simulink model "Manipulator_Power_Simulink1"  (R2021b)
settings: Solver=VariableStepAuto  StartTime=0.0  StopTime=10.0  RelTol=1e-3
libraries: fl_lib x72, fl_ps_legacy_lib x32, nesl_utility x24, ee_lib x8, simulink x4, slpidlib x4, simulink_extras x4
(part 2 of 2)

== system Manipulator_Power_Simulink1/JOINT2/Controller/Speed ==
  Ref : Inport  RequirementInfo={} %GIDa_133d2fbd_c93e_4f77_b4ac_eab9d76c42d5
  ERef : fl_lib/Electrical/Electrical Elements/Electrical Reference  RequirementInfo={} %GIDa_7d76ed12_3202_4e07_9a81_a49e1b94768a
  Step Rate and Direction : Subsystem  RequirementInfo={} %GIDa_caaf0cf5_7010_465f_9918_d7533aa9d66e
  Voltage-Controlled Pulse Generator : Subsystem  RequirementInfo={} %GIDa_c6184c00_e7ae_4ed6_b023_dd2e423edd06
  PWM : PMIOPort  RequirementInfo={} %GIDa_212c39cb_5b57_476e_a698_4d1e9cdd5427  Side=Right
  0v : PMIOPort  RequirementInfo={} %GIDa_c3c92952_d7df_46f2_a6c1_61685cd34345  Port=2  Side=Right
  REV : PMIOPort  RequirementInfo={} %GIDa_dc8a3b62_1286_4359_8672_6bb9b44ae351  Port=3  Side=Right
  wires:
  Ref/1 -> Step Rate and Direction/1(Reference)
  connections:
  PWM/RConn1 -- Voltage-Controlled Pulse Generator/RConn1
  Voltage-Controlled Pulse Generator/RConn2 -- 0v/RConn1 -- ERef/LConn1
  Step Rate and Direction/RConn1 -- REV/RConn1
  Step Rate and Direction/RConn2 -- Voltage-Controlled Pulse Generator/LConn1

== system Manipulator_Power_Simulink1/JOINT3/Controller/Speed ==
  Ref : Inport  RequirementInfo={} %GIDa_816022ef_432a_4a79_90a7_2ae6cbd59fcd
  ERef : fl_lib/Electrical/Electrical Elements/Electrical Reference  RequirementInfo={} %GIDa_196008e7_2150_4d1c_9562_2b404e1eb384
  Step Rate and Direction : Subsystem  RequirementInfo={} %GIDa_3dc02a5d_9463_4040_a7f9_8c5ed42feb4d
  Voltage-Controlled Pulse Generator : Subsystem  RequirementInfo={} %GIDa_cda5a4f7_7bce_4a17_92d2_0249b497aa56
  PWM : PMIOPort  RequirementInfo={} %GIDa_ae6e6dfd_0883_41b5_a79f_f2a88b9bb8a5  Side=Right
  0v : PMIOPort  RequirementInfo={} %GIDa_84d0f212_669f_417f_b7e6_49da8841d292  Port=2  Side=Right
  REV : PMIOPort  RequirementInfo={} %GIDa_363b8ad7_587b_486d_9c01_9ecb04e88f52  Port=3  Side=Right
  wires:
  Ref/1 -> Step Rate and Direction/1(Reference)
  connections:
  Step Rate and Direction/RConn2 -- Voltage-Controlled Pulse Generator/LConn1
  Step Rate and Direction/RConn1 -- REV/RConn1
  ERef/LConn1 -- 0v/RConn1 -- Voltage-Controlled Pulse Generator/RConn2
  PWM/RConn1 -- Voltage-Controlled Pulse Generator/RConn1

== system Manipulator_Power_Simulink1/JOINT4/Controller/Speed ==
  Ref : Inport  RequirementInfo={} %GIDa_d717e889_664f_4dd2_8736_eb6c370576c8
  ERef : fl_lib/Electrical/Electrical Elements/Electrical Reference  RequirementInfo={} %GIDa_8f4f37d8_c331_48d0_9e36_178249331710
  Step Rate and Direction : Subsystem  RequirementInfo={} %GIDa_7f64dba6_34d7_4fd6_b7e6_8ef2aa4dbaeb
  Voltage-Controlled Pulse Generator : Subsystem  RequirementInfo={} %GIDa_cf4eb0bf_28be_416a_a242_a03039ffa540
  PWM : PMIOPort  RequirementInfo={} %GIDa_aef454f5_c686_4161_86a7_873aeed7fd4b  Side=Right
  0v : PMIOPort  RequirementInfo={} %GIDa_3be3be1f_d3f7_46ea_ae96_b67254762afc  Port=2  Side=Right
  REV : PMIOPort  RequirementInfo={} %GIDa_ffa23ca5_42c1_4813_9242_4a9203d3890b  Port=3  Side=Right
  wires:
  Ref/1 -> Step Rate and Direction/1(Reference)
  connections:
  PWM/RConn1 -- Voltage-Controlled Pulse Generator/RConn1
  Voltage-Controlled Pulse Generator/RConn2 -- 0v/RConn1 -- ERef/LConn1
  Step Rate and Direction/RConn1 -- REV/RConn1
  Step Rate and Direction/RConn2 -- Voltage-Controlled Pulse Generator/LConn1

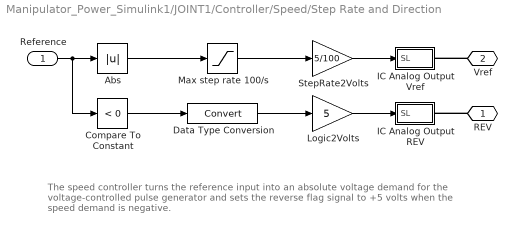
== system Manipulator_Power_Simulink1/JOINT1/Controller/Speed/Step Rate and Direction ==
  note: The speed controller turns the reference input into an absolute voltage demand for the
      | voltage-controlled pulse generator and sets the reverse flag signal to +5 volts when the
      | speed demand is negative.
  Reference : Inport  RequirementInfo={} %GIDa_a4d0a8f3_775c_42b8_9ce6_c57082dd7fd6
  Abs : Abs  RequirementInfo={} %GIDa_7613da56_6ee1_41bb_bf24_79eccb83e254
  Compare To Constant : simulink/Logic and Bit Operations/Compare To Constant  relop=<  const=0  OutDataTypeStr=uint8  ZeroCross=off
  Data Type Conversion : DataTypeConversion  RequirementInfo={} %GIDa_15417bf0_c7ec_4a8f_8ffd_c88ebbfd43ea
  IC Analog Output REV : Subsystem  RequirementInfo={} %GIDa_2381db1b_a9cd_4814_b69d_fad528507182
  IC Analog Output Vref : Subsystem  RequirementInfo={} %GIDa_7a2ed817_81c4_46ea_bee9_8975aad226ea
  Logic2Volts : Gain  RequirementInfo={} %GIDa_359c6216_a839_4c16_a394_d78c702d9162  Gain=5
  Max step rate 100/s : Saturate  RequirementInfo={} %GIDa_432da2a1_418c_4d16_83eb_56a19b9fecce  UpperLimit=100  LowerLimit=0
  StepRate2Volts : Gain  RequirementInfo={} %GIDa_aa390892_47b5_48bb_8fe1_8b1239142bf5  Gain=5/100
  REV : PMIOPort  RequirementInfo={} %GIDa_b21a2a82_f1de_4c93_a224_afadd27e55c2  Side=Right
  Vref : PMIOPort  RequirementInfo={} %GIDa_5a2899ae_9d44_4071_a42f_9f02a65277c8  Port=2  Side=Right
  wires:
  Logic2Volts/1 -> IC Analog Output REV/1(SL)
  Abs/1 -> Max step rate 100/s/1
  Reference/1 -> Abs/1, Compare To Constant/1
  Compare To Constant/1 -> Data Type Conversion/1
  Data Type Conversion/1 -> Logic2Volts/1
  Max step rate 100/s/1 -> StepRate2Volts/1
  StepRate2Volts/1 -> IC Analog Output Vref/1(SL)
  connections:
  Vref/RConn1 -- IC Analog Output Vref/RConn1
  REV/RConn1 -- IC Analog Output REV/RConn1

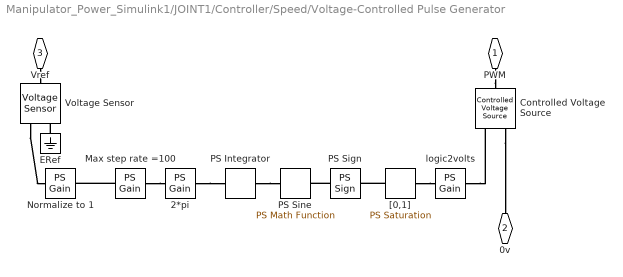
== system Manipulator_Power_Simulink1/JOINT1/Controller/Speed/Voltage-Controlled Pulse Generator ==
  2*pi : fl_ps_legacy_lib/Legacy Physical Signals/Functions/PS Gain  RequirementInfo={} %GIDa_61df0c9e_b235_4c70_930a_adc0727db65f  gain=-2*pi
  Controlled Voltage Source : fl_lib/Electrical/Electrical Sources/Controlled Voltage Source  RequirementInfo={} %GIDa_890246c1_4e7d_432c_91b9_002d9def5f11
  ERef : fl_lib/Electrical/Electrical Elements/Electrical Reference  RequirementInfo={} %GIDa_3d71df36_8a4a_4c67_937d_640ca4b360d2
  Max step rate =100 : fl_ps_legacy_lib/Legacy Physical Signals/Functions/PS Gain  RequirementInfo={} %GIDa_eb934f0b_f6ff_49ce_bc85_53990e09ede5  gain=100
  Normalize to 1 : fl_ps_legacy_lib/Legacy Physical Signals/Functions/PS Gain  RequirementInfo={} %GIDa_5c71ac23_9195_42cc_b2ed_1502285f8c0f  gain=1/5
  PS Integrator : fl_ps_legacy_lib/Legacy Physical Signals/Linear Operators/PS Integrator  RequirementInfo={} %GIDa_2c83dace_df5d_4329_b79b_3a0dcf4e6b2a  x0=0
      settings: SourceProductBaseCode=SS  InternalSimscapePortConfiguration="{\"Bottom\":[],\"Left\":[{\"id\":\"I\",\"label\":\"\",\"type\":\"input\"}],\"Right\":[{\"id\":\"O\",\"label\":\"\",\"type\":\"output\"}],\"Top\":[]}"
  PS Sign : fl_ps_legacy_lib/Legacy Physical Signals/Nonlinear Operators/PS Sign  RequirementInfo={} %GIDa_f0cac072_c839_41db_b2f7_6ab4e4664324
      settings: SourceProductBaseCode=SS  InternalSimscapePortConfiguration="{\"Bottom\":[],\"Left\":[{\"id\":\"I\",\"label\":\"\",\"type\":\"input\"}],\"Right\":[{\"id\":\"O\",\"label\":\"\",\"type\":\"output\"}],\"Top\":[]}"
  PS Sine : fl_ps_legacy_lib/Legacy Physical Signals/Functions/PS Math Function  RequirementInfo={} %GIDa_6e5c4b4c_1fe3_442e_b21e_5b744a8abd76  fcn_choice=1
      settings: SourceProductBaseCode=SS  InternalSimscapePortConfiguration="{\"Bottom\":[],\"Left\":[{\"id\":\"I\",\"label\":\"\",\"type\":\"input\"}],\"Right\":[{\"id\":\"O\",\"label\":\"\",\"type\":\"output\"}],\"Top\":[]}"
  Voltage Sensor : fl_lib/Electrical/Electrical Sensors/Voltage Sensor  RequirementInfo={} %GIDa_a373e7ac_be28_43af_8d8c_244c39e826c1
  "[0,1]" : fl_ps_legacy_lib/Legacy Physical Signals/Nonlinear Operators/PS Saturation  RequirementInfo={} %GIDa_5495923a_3b44_4237_bdb7_0f954ea1e40d  upper_limit=1  lower_limit=0
      settings: SourceProductBaseCode=SS  InternalSimscapePortConfiguration="{\"Bottom\":[],\"Left\":[{\"id\":\"I\",\"label\":\"\",\"type\":\"input\"}],\"Right\":[{\"id\":\"O\",\"label\":\"\",\"type\":\"output\"}],\"Top\":[]}"
  logic2volts : fl_ps_legacy_lib/Legacy Physical Signals/Functions/PS Gain  RequirementInfo={} %GIDa_083ec3bc_2847_48bb_b782_91084d8168f5  gain=5
  PWM : PMIOPort  RequirementInfo={} %GIDa_4cd06a5c_1eea_49eb_bdb7_282e6aefe270  Side=Right
  0v : PMIOPort  RequirementInfo={} %GIDa_96d2d6b6_c14e_4d63_87b4_9d47c63deab9  Port=2  Side=Right
  Vref : PMIOPort  RequirementInfo={} %GIDa_2a267a3e_713f_4133_af62_9dc00d10e885  Port=3  Side=Left
  connections:
  logic2volts/RConn1 -- Controlled Voltage Source/RConn1
  "[0,1]"/RConn1 -- logic2volts/LConn1
  "[0,1]"/LConn1 -- PS Sign/RConn1
  PS Sign/LConn1 -- PS Sine/RConn1
  PS Integrator/RConn1 -- PS Sine/LConn1
  2*pi/RConn1 -- PS Integrator/LConn1
  Max step rate =100/RConn1 -- 2*pi/LConn1
  Max step rate =100/LConn1 -- Normalize to 1/RConn1
  Voltage Sensor/RConn1 -- Normalize to 1/LConn1
  ERef/LConn1 -- Voltage Sensor/RConn2
  Vref/RConn1 -- Voltage Sensor/LConn1
  Controlled Voltage Source/RConn2 -- 0v/RConn1
  PWM/RConn1 -- Controlled Voltage Source/LConn1

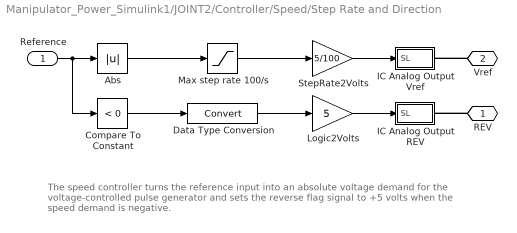
== system Manipulator_Power_Simulink1/JOINT2/Controller/Speed/Step Rate and Direction ==
  note: The speed controller turns the reference input into an absolute voltage demand for the
      | voltage-controlled pulse generator and sets the reverse flag signal to +5 volts when the
      | speed demand is negative.
  Reference : Inport  RequirementInfo={} %GIDa_90aba829_d451_4a5e_aa85_55f83649f4db
  Abs : Abs  RequirementInfo={} %GIDa_c9b203d5_6184_4a9d_ad90_f83fc17c6376
  Compare To Constant : simulink/Logic and Bit Operations/Compare To Constant  relop=<  const=0  OutDataTypeStr=uint8  ZeroCross=off
  Data Type Conversion : DataTypeConversion  RequirementInfo={} %GIDa_43c8ecc9_fa97_4981_9627_7cee22fda550
  IC Analog Output REV : Subsystem  RequirementInfo={} %GIDa_ece9aa21_0efe_49d4_b00f_8f3649ea2b46
  IC Analog Output Vref : Subsystem  RequirementInfo={} %GIDa_c052096d_f211_49fe_bd90_0695814d8abb
  Logic2Volts : Gain  RequirementInfo={} %GIDa_66d68ea1_9468_4636_a012_2b3722893939  Gain=5
  Max step rate 100/s : Saturate  RequirementInfo={} %GIDa_e4ccdf5f_c923_46ec_be92_c720fdfcfe89  UpperLimit=100  LowerLimit=0
  StepRate2Volts : Gain  RequirementInfo={} %GIDa_d1820e5c_7501_48ce_a768_ecf098b9c526  Gain=5/100
  REV : PMIOPort  RequirementInfo={} %GIDa_0581cefe_2bd8_489e_9052_9096d03c1b9a  Side=Right
  Vref : PMIOPort  RequirementInfo={} %GIDa_241c3493_720f_4f49_b456_999d10fd9f84  Port=2  Side=Right
  wires:
  StepRate2Volts/1 -> IC Analog Output Vref/1(SL)
  Max step rate 100/s/1 -> StepRate2Volts/1
  Data Type Conversion/1 -> Logic2Volts/1
  Compare To Constant/1 -> Data Type Conversion/1
  Reference/1 -> Compare To Constant/1, Abs/1
  Abs/1 -> Max step rate 100/s/1
  Logic2Volts/1 -> IC Analog Output REV/1(SL)
  connections:
  REV/RConn1 -- IC Analog Output REV/RConn1
  Vref/RConn1 -- IC Analog Output Vref/RConn1

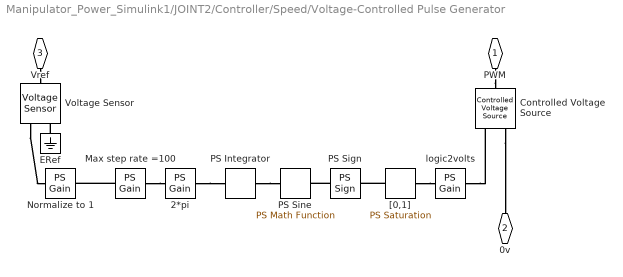
== system Manipulator_Power_Simulink1/JOINT2/Controller/Speed/Voltage-Controlled Pulse Generator ==
  2*pi : fl_ps_legacy_lib/Legacy Physical Signals/Functions/PS Gain  RequirementInfo={} %GIDa_39e0f13f_ed03_40b4_bff0_704818bbd013  gain=-2*pi
  Controlled Voltage Source : fl_lib/Electrical/Electrical Sources/Controlled Voltage Source  RequirementInfo={} %GIDa_3f254ddd_a112_40da_8740_ab4ae00e6674
  ERef : fl_lib/Electrical/Electrical Elements/Electrical Reference  RequirementInfo={} %GIDa_aa12cf46_d350_4702_8bd6_c00e57a06f4e
  Max step rate =100 : fl_ps_legacy_lib/Legacy Physical Signals/Functions/PS Gain  RequirementInfo={} %GIDa_0262f2d3_1b67_4f1f_8188_fa8785035f93  gain=100
  Normalize to 1 : fl_ps_legacy_lib/Legacy Physical Signals/Functions/PS Gain  RequirementInfo={} %GIDa_8dc38732_8c04_47cc_b45a_cab155dda67b  gain=1/5
  PS Integrator : fl_ps_legacy_lib/Legacy Physical Signals/Linear Operators/PS Integrator  RequirementInfo={} %GIDa_51806525_f935_4d2f_8466_5852c52c21b4  x0=0
      settings: SourceProductBaseCode=SS  InternalSimscapePortConfiguration="{\"Bottom\":[],\"Left\":[{\"id\":\"I\",\"label\":\"\",\"type\":\"input\"}],\"Right\":[{\"id\":\"O\",\"label\":\"\",\"type\":\"output\"}],\"Top\":[]}"
  PS Sign : fl_ps_legacy_lib/Legacy Physical Signals/Nonlinear Operators/PS Sign  RequirementInfo={} %GIDa_979e4ac6_6728_4e81_892d_596687daac1f
      settings: SourceProductBaseCode=SS  InternalSimscapePortConfiguration="{\"Bottom\":[],\"Left\":[{\"id\":\"I\",\"label\":\"\",\"type\":\"input\"}],\"Right\":[{\"id\":\"O\",\"label\":\"\",\"type\":\"output\"}],\"Top\":[]}"
  PS Sine : fl_ps_legacy_lib/Legacy Physical Signals/Functions/PS Math Function  RequirementInfo={} %GIDa_d7491fba_bca0_4560_8f49_912ad2ea4dc1  fcn_choice=1
      settings: SourceProductBaseCode=SS  InternalSimscapePortConfiguration="{\"Bottom\":[],\"Left\":[{\"id\":\"I\",\"label\":\"\",\"type\":\"input\"}],\"Right\":[{\"id\":\"O\",\"label\":\"\",\"type\":\"output\"}],\"Top\":[]}"
  Voltage Sensor : fl_lib/Electrical/Electrical Sensors/Voltage Sensor  RequirementInfo={} %GIDa_d2de3142_6796_463e_b13f_d7b525af65fd
  "[0,1]" : fl_ps_legacy_lib/Legacy Physical Signals/Nonlinear Operators/PS Saturation  RequirementInfo={} %GIDa_2a538ce2_d55b_4ca7_b3f2_8996148affe4  upper_limit=1  lower_limit=0
      settings: SourceProductBaseCode=SS  InternalSimscapePortConfiguration="{\"Bottom\":[],\"Left\":[{\"id\":\"I\",\"label\":\"\",\"type\":\"input\"}],\"Right\":[{\"id\":\"O\",\"label\":\"\",\"type\":\"output\"}],\"Top\":[]}"
  logic2volts : fl_ps_legacy_lib/Legacy Physical Signals/Functions/PS Gain  RequirementInfo={} %GIDa_1da96181_0729_44e5_ab12_b3f446b1ef09  gain=5
  PWM : PMIOPort  RequirementInfo={} %GIDa_5ea3616d_b8a3_4cc2_9d21_4ee89ba264a6  Side=Right
  0v : PMIOPort  RequirementInfo={} %GIDa_217c9688_de14_4ae3_9fb7_afb5736173ab  Port=2  Side=Right
  Vref : PMIOPort  RequirementInfo={} %GIDa_a8697067_ee00_4349_a0d9_3a9618a53fc4  Port=3  Side=Left
  connections:
  PWM/RConn1 -- Controlled Voltage Source/LConn1
  Controlled Voltage Source/RConn2 -- 0v/RConn1
  Vref/RConn1 -- Voltage Sensor/LConn1
  ERef/LConn1 -- Voltage Sensor/RConn2
  Voltage Sensor/RConn1 -- Normalize to 1/LConn1
  Max step rate =100/LConn1 -- Normalize to 1/RConn1
  Max step rate =100/RConn1 -- 2*pi/LConn1
  2*pi/RConn1 -- PS Integrator/LConn1
  PS Integrator/RConn1 -- PS Sine/LConn1
  PS Sign/LConn1 -- PS Sine/RConn1
  "[0,1]"/LConn1 -- PS Sign/RConn1
  "[0,1]"/RConn1 -- logic2volts/LConn1
  logic2volts/RConn1 -- Controlled Voltage Source/RConn1

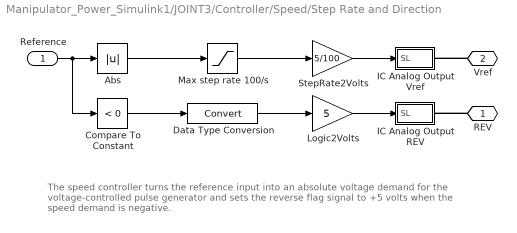
== system Manipulator_Power_Simulink1/JOINT3/Controller/Speed/Step Rate and Direction ==
  note: The speed controller turns the reference input into an absolute voltage demand for the
      | voltage-controlled pulse generator and sets the reverse flag signal to +5 volts when the
      | speed demand is negative.
  Reference : Inport  RequirementInfo={} %GIDa_e41558cf_4cf6_4664_8058_0312b625df14
  Abs : Abs  RequirementInfo={} %GIDa_35eed948_d26b_445f_bafd_d904c0444c28
  Compare To Constant : simulink/Logic and Bit Operations/Compare To Constant  relop=<  const=0  OutDataTypeStr=uint8  ZeroCross=off
  Data Type Conversion : DataTypeConversion  RequirementInfo={} %GIDa_c55a0244_950d_4825_8ab4_38179d1a507b
  IC Analog Output REV : Subsystem  RequirementInfo={} %GIDa_b1afa9ee_bd98_4eaf_a4b6_2b4cd345befe
  IC Analog Output Vref : Subsystem  RequirementInfo={} %GIDa_dc1860ae_6cf6_4062_b3c0_bc69cd577efa
  Logic2Volts : Gain  RequirementInfo={} %GIDa_797ab312_e620_4b9d_a3cb_83908b24325f  Gain=5
  Max step rate 100/s : Saturate  RequirementInfo={} %GIDa_b28a9105_40d4_4f94_b332_87ddbf6cc823  UpperLimit=100  LowerLimit=0
  StepRate2Volts : Gain  RequirementInfo={} %GIDa_33a0acae_85f0_4059_9e4d_70e14c1e9ee0  Gain=5/100
  REV : PMIOPort  RequirementInfo={} %GIDa_933b063f_5666_4fd7_a8e4_d5d0fda9cf01  Side=Right
  Vref : PMIOPort  RequirementInfo={} %GIDa_5cb1fd0e_612c_4f03_ad27_996cba0e183e  Port=2  Side=Right
  wires:
  Logic2Volts/1 -> IC Analog Output REV/1(SL)
  Abs/1 -> Max step rate 100/s/1
  Reference/1 -> Abs/1, Compare To Constant/1
  Compare To Constant/1 -> Data Type Conversion/1
  Data Type Conversion/1 -> Logic2Volts/1
  Max step rate 100/s/1 -> StepRate2Volts/1
  StepRate2Volts/1 -> IC Analog Output Vref/1(SL)
  connections:
  Vref/RConn1 -- IC Analog Output Vref/RConn1
  REV/RConn1 -- IC Analog Output REV/RConn1

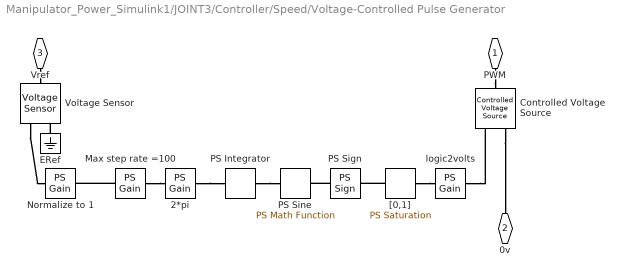
== system Manipulator_Power_Simulink1/JOINT3/Controller/Speed/Voltage-Controlled Pulse Generator ==
  2*pi : fl_ps_legacy_lib/Legacy Physical Signals/Functions/PS Gain  RequirementInfo={} %GIDa_b740e3cc_25e5_4f30_a797_9c6ce1231883  gain=-2*pi
  Controlled Voltage Source : fl_lib/Electrical/Electrical Sources/Controlled Voltage Source  RequirementInfo={} %GIDa_79ae19dc_ab4d_4dc5_8ad2_a3820feb6f8a
  ERef : fl_lib/Electrical/Electrical Elements/Electrical Reference  RequirementInfo={} %GIDa_a7b81ec0_8f1c_4f37_946e_7c8db6e35412
  Max step rate =100 : fl_ps_legacy_lib/Legacy Physical Signals/Functions/PS Gain  RequirementInfo={} %GIDa_9cbbd355_74fa_4684_bd10_e89996d8b818  gain=100
  Normalize to 1 : fl_ps_legacy_lib/Legacy Physical Signals/Functions/PS Gain  RequirementInfo={} %GIDa_6a0b4414_d6fe_414b_a7ee_e9952919e3b0  gain=1/5
  PS Integrator : fl_ps_legacy_lib/Legacy Physical Signals/Linear Operators/PS Integrator  RequirementInfo={} %GIDa_861ac414_fd0d_4e43_aab2_71d62cf93405  x0=0
      settings: SourceProductBaseCode=SS  InternalSimscapePortConfiguration="{\"Bottom\":[],\"Left\":[{\"id\":\"I\",\"label\":\"\",\"type\":\"input\"}],\"Right\":[{\"id\":\"O\",\"label\":\"\",\"type\":\"output\"}],\"Top\":[]}"
  PS Sign : fl_ps_legacy_lib/Legacy Physical Signals/Nonlinear Operators/PS Sign  RequirementInfo={} %GIDa_0be84da2_46c6_4942_8052_a17cc1d925c5
      settings: SourceProductBaseCode=SS  InternalSimscapePortConfiguration="{\"Bottom\":[],\"Left\":[{\"id\":\"I\",\"label\":\"\",\"type\":\"input\"}],\"Right\":[{\"id\":\"O\",\"label\":\"\",\"type\":\"output\"}],\"Top\":[]}"
  PS Sine : fl_ps_legacy_lib/Legacy Physical Signals/Functions/PS Math Function  RequirementInfo={} %GIDa_7faa4cb9_08e4_49ad_90c8_4ace7a404225  fcn_choice=1
      settings: SourceProductBaseCode=SS  InternalSimscapePortConfiguration="{\"Bottom\":[],\"Left\":[{\"id\":\"I\",\"label\":\"\",\"type\":\"input\"}],\"Right\":[{\"id\":\"O\",\"label\":\"\",\"type\":\"output\"}],\"Top\":[]}"
  Voltage Sensor : fl_lib/Electrical/Electrical Sensors/Voltage Sensor  RequirementInfo={} %GIDa_17c2efd4_9685_4d35_9a32_364b52e641a9
  "[0,1]" : fl_ps_legacy_lib/Legacy Physical Signals/Nonlinear Operators/PS Saturation  RequirementInfo={} %GIDa_279308bb_61ee_4a77_99bb_4cc027ccbb41  upper_limit=1  lower_limit=0
      settings: SourceProductBaseCode=SS  InternalSimscapePortConfiguration="{\"Bottom\":[],\"Left\":[{\"id\":\"I\",\"label\":\"\",\"type\":\"input\"}],\"Right\":[{\"id\":\"O\",\"label\":\"\",\"type\":\"output\"}],\"Top\":[]}"
  logic2volts : fl_ps_legacy_lib/Legacy Physical Signals/Functions/PS Gain  RequirementInfo={} %GIDa_2e4f5c9e_e808_4ed4_bda1_44483ff0252e  gain=5
  PWM : PMIOPort  RequirementInfo={} %GIDa_0ffd18b3_a9dd_40a7_b8a8_1eb886078c4b  Side=Right
  0v : PMIOPort  RequirementInfo={} %GIDa_ebf6917d_3fbc_409e_92ca_a4843bad0fc7  Port=2  Side=Right
  Vref : PMIOPort  RequirementInfo={} %GIDa_eb93b3dc_32ae_432d_9f8e_911f11189326  Port=3  Side=Left
  connections:
  logic2volts/RConn1 -- Controlled Voltage Source/RConn1
  "[0,1]"/RConn1 -- logic2volts/LConn1
  "[0,1]"/LConn1 -- PS Sign/RConn1
  PS Sign/LConn1 -- PS Sine/RConn1
  PS Integrator/RConn1 -- PS Sine/LConn1
  2*pi/RConn1 -- PS Integrator/LConn1
  Max step rate =100/RConn1 -- 2*pi/LConn1
  Max step rate =100/LConn1 -- Normalize to 1/RConn1
  Voltage Sensor/RConn1 -- Normalize to 1/LConn1
  ERef/LConn1 -- Voltage Sensor/RConn2
  Vref/RConn1 -- Voltage Sensor/LConn1
  Controlled Voltage Source/RConn2 -- 0v/RConn1
  PWM/RConn1 -- Controlled Voltage Source/LConn1

== system Manipulator_Power_Simulink1/JOINT4/Controller/Speed/Step Rate and Direction ==
  note: The speed controller turns the reference input into an absolute voltage demand for the
      | voltage-controlled pulse generator and sets the reverse flag signal to +5 volts when the
      | speed demand is negative.
  Reference : Inport  RequirementInfo={} %GIDa_3c1cf7f4_8aab_4b27_a15c_4f3445e2c108
  Abs : Abs  RequirementInfo={} %GIDa_a4c5ff9f_f4bc_4419_b386_0b71cd9cee93
  Compare To Constant : simulink/Logic and Bit Operations/Compare To Constant  relop=<  const=0  OutDataTypeStr=uint8  ZeroCross=off
  Data Type Conversion : DataTypeConversion  RequirementInfo={} %GIDa_4f1de8ed_cf8e_4042_831c_225004c8baf2
  IC Analog Output REV : Subsystem  RequirementInfo={} %GIDa_5777efa7_63e1_4053_84f0_4436bc30bc7b
  IC Analog Output Vref : Subsystem  RequirementInfo={} %GIDa_a7a73a31_6963_4ebd_8f5f_7274d19066b4
  Logic2Volts : Gain  RequirementInfo={} %GIDa_5f42dbbb_8cbc_46eb_b421_9f975a17c297  Gain=5
  Max step rate 100/s : Saturate  RequirementInfo={} %GIDa_95e6a340_9705_4d91_b485_31b055d80ecd  UpperLimit=100  LowerLimit=0
  StepRate2Volts : Gain  RequirementInfo={} %GIDa_b37e94c9_8c2e_41ef_a5c1_e1e9e4ddc3ce  Gain=5/100
  REV : PMIOPort  RequirementInfo={} %GIDa_7dc94042_af75_405a_a6d0_8ac37ce84735  Side=Right
  Vref : PMIOPort  RequirementInfo={} %GIDa_2d157ce9_f094_4672_bc4f_925f4b8a320b  Port=2  Side=Right
  wires:
  StepRate2Volts/1 -> IC Analog Output Vref/1(SL)
  Max step rate 100/s/1 -> StepRate2Volts/1
  Data Type Conversion/1 -> Logic2Volts/1
  Compare To Constant/1 -> Data Type Conversion/1
  Reference/1 -> Compare To Constant/1, Abs/1
  Abs/1 -> Max step rate 100/s/1
  Logic2Volts/1 -> IC Analog Output REV/1(SL)
  connections:
  REV/RConn1 -- IC Analog Output REV/RConn1
  Vref/RConn1 -- IC Analog Output Vref/RConn1

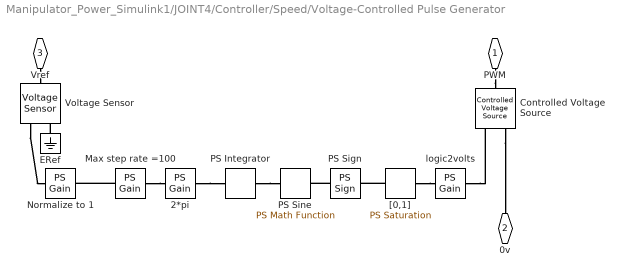
== system Manipulator_Power_Simulink1/JOINT4/Controller/Speed/Voltage-Controlled Pulse Generator ==
  2*pi : fl_ps_legacy_lib/Legacy Physical Signals/Functions/PS Gain  RequirementInfo={} %GIDa_66813b41_8fd0_4aca_b763_be0e326a44b9  gain=-2*pi
  Controlled Voltage Source : fl_lib/Electrical/Electrical Sources/Controlled Voltage Source  RequirementInfo={} %GIDa_65cba9e0_ee6d_4148_b9d1_3429b3ec2b17
  ERef : fl_lib/Electrical/Electrical Elements/Electrical Reference  RequirementInfo={} %GIDa_cddc951d_b424_40ff_9103_14f4b3e43b41
  Max step rate =100 : fl_ps_legacy_lib/Legacy Physical Signals/Functions/PS Gain  RequirementInfo={} %GIDa_ba40341b_bcb9_408b_afc4_04d5e290f9fe  gain=100
  Normalize to 1 : fl_ps_legacy_lib/Legacy Physical Signals/Functions/PS Gain  RequirementInfo={} %GIDa_5d235928_9757_4d05_9898_0539ebf6ac7e  gain=1/5
  PS Integrator : fl_ps_legacy_lib/Legacy Physical Signals/Linear Operators/PS Integrator  RequirementInfo={} %GIDa_46c26e47_d25d_4678_9c77_a70f260d309f  x0=0
      settings: SourceProductBaseCode=SS  InternalSimscapePortConfiguration="{\"Bottom\":[],\"Left\":[{\"id\":\"I\",\"label\":\"\",\"type\":\"input\"}],\"Right\":[{\"id\":\"O\",\"label\":\"\",\"type\":\"output\"}],\"Top\":[]}"
  PS Sign : fl_ps_legacy_lib/Legacy Physical Signals/Nonlinear Operators/PS Sign  RequirementInfo={} %GIDa_90bbde27_a939_4f52_8f32_954059597cda
      settings: SourceProductBaseCode=SS  InternalSimscapePortConfiguration="{\"Bottom\":[],\"Left\":[{\"id\":\"I\",\"label\":\"\",\"type\":\"input\"}],\"Right\":[{\"id\":\"O\",\"label\":\"\",\"type\":\"output\"}],\"Top\":[]}"
  PS Sine : fl_ps_legacy_lib/Legacy Physical Signals/Functions/PS Math Function  RequirementInfo={} %GIDa_fe48fc95_b233_4a8d_92fb_2e7595bfc7f9  fcn_choice=1
      settings: SourceProductBaseCode=SS  InternalSimscapePortConfiguration="{\"Bottom\":[],\"Left\":[{\"id\":\"I\",\"label\":\"\",\"type\":\"input\"}],\"Right\":[{\"id\":\"O\",\"label\":\"\",\"type\":\"output\"}],\"Top\":[]}"
  Voltage Sensor : fl_lib/Electrical/Electrical Sensors/Voltage Sensor  RequirementInfo={} %GIDa_f6a543b8_fe6d_4c52_ba0d_d5dd69f7b865
  "[0,1]" : fl_ps_legacy_lib/Legacy Physical Signals/Nonlinear Operators/PS Saturation  RequirementInfo={} %GIDa_c0b3b3c9_3657_471f_ac15_3fc2c11f2843  upper_limit=1  lower_limit=0
      settings: SourceProductBaseCode=SS  InternalSimscapePortConfiguration="{\"Bottom\":[],\"Left\":[{\"id\":\"I\",\"label\":\"\",\"type\":\"input\"}],\"Right\":[{\"id\":\"O\",\"label\":\"\",\"type\":\"output\"}],\"Top\":[]}"
  logic2volts : fl_ps_legacy_lib/Legacy Physical Signals/Functions/PS Gain  RequirementInfo={} %GIDa_8f360269_0cb4_481d_b6f5_c992905e9f39  gain=5
  PWM : PMIOPort  RequirementInfo={} %GIDa_6e010553_9f83_4703_a732_cd3f866b258e  Side=Right
  0v : PMIOPort  RequirementInfo={} %GIDa_cfc93a1d_2cc5_43ca_af35_a8fdc155dd0d  Port=2  Side=Right
  Vref : PMIOPort  RequirementInfo={} %GIDa_330d7adb_35be_4f9a_92d8_c21dff02abe9  Port=3  Side=Left
  connections:
  PWM/RConn1 -- Controlled Voltage Source/LConn1
  Controlled Voltage Source/RConn2 -- 0v/RConn1
  Vref/RConn1 -- Voltage Sensor/LConn1
  ERef/LConn1 -- Voltage Sensor/RConn2
  Voltage Sensor/RConn1 -- Normalize to 1/LConn1
  Max step rate =100/LConn1 -- Normalize to 1/RConn1
  Max step rate =100/RConn1 -- 2*pi/LConn1
  2*pi/RConn1 -- PS Integrator/LConn1
  PS Integrator/RConn1 -- PS Sine/LConn1
  PS Sign/LConn1 -- PS Sine/RConn1
  "[0,1]"/LConn1 -- PS Sign/RConn1
  "[0,1]"/RConn1 -- logic2volts/LConn1
  logic2volts/RConn1 -- Controlled Voltage Source/RConn1

== system Manipulator_Power_Simulink1/JOINT1/Controller/Speed/Step Rate and Direction/IC Analog Output REV ==
  SL : Inport  RequirementInfo={} %GIDa_02c26200_b0a8_4d42_bf0d_0515453987ae
  Controlled Voltage Source : fl_lib/Electrical/Electrical Sources/Controlled Voltage Source  RequirementInfo={} %GIDa_0c5eaec1_3691_4fd4_aa27_3131dd8f70af
  ERef : fl_lib/Electrical/Electrical Elements/Electrical Reference  RequirementInfo={} %GIDa_7b4c6f4b_a7ad_4dd6_b0e2_f0e6e1e68a66
  Simulink-PS Converter : nesl_utility/Simulink-PS Converter  RequirementInfo={} %GIDa_24446364_eec0_4d48_8623_babd559e7409  PhysicalDomain=network_engine_domain  SubClassName=ps_input  LeftPortType=input  RightPortType=output  PseudoPeriodic=off  Frequencies=[]  NoiseDistribution=none  NoiseParameters=[]  Unit=V  AffineConversion=off  FilteringAndDerivatives=zero  SimscapeFilterOrder=1  InputFilterTimeConstant=.001  UdotUserProvided=0
      settings: SourceProductBaseCode=PW,SS
  V : PMIOPort  RequirementInfo={} %GIDa_c38a79aa_0966_4c84_b0e1_9462a22e10f8  Side=Right
  wires:
  SL/1 -> Simulink-PS Converter/1
  connections:
  ERef/LConn1 -- Controlled Voltage Source/RConn2
  V/RConn1 -- Controlled Voltage Source/LConn1
  Simulink-PS Converter/RConn1 -- Controlled Voltage Source/RConn1

== system Manipulator_Power_Simulink1/JOINT1/Controller/Speed/Step Rate and Direction/IC Analog Output Vref ==
  SL : Inport  RequirementInfo={} %GIDa_f1190acc_3ebd_43d4_99b6_97e9d6f492b0
  Controlled Voltage Source : fl_lib/Electrical/Electrical Sources/Controlled Voltage Source  RequirementInfo={} %GIDa_8b110c0c_63b4_4b21_950a_268b6b8bab3d
  ERef : fl_lib/Electrical/Electrical Elements/Electrical Reference  RequirementInfo={} %GIDa_b02017e9_721d_4b2d_986b_adb6afa2a9d3
  Simulink-PS Converter : nesl_utility/Simulink-PS Converter  RequirementInfo={} %GIDa_e31afa12_1f43_4fe4_975f_f7db0b5afe35  PhysicalDomain=network_engine_domain  SubClassName=ps_input  LeftPortType=input  RightPortType=output  PseudoPeriodic=off  Frequencies=[]  NoiseDistribution=none  NoiseParameters=[]  Unit=V  AffineConversion=off  FilteringAndDerivatives=zero  SimscapeFilterOrder=1  InputFilterTimeConstant=.001  UdotUserProvided=0
      settings: SourceProductBaseCode=PW,SS
  V : PMIOPort  RequirementInfo={} %GIDa_7fc42ce3_83a4_46fe_bd47_de0850ef379b  Side=Right
  wires:
  SL/1 -> Simulink-PS Converter/1
  connections:
  Simulink-PS Converter/RConn1 -- Controlled Voltage Source/RConn1
  V/RConn1 -- Controlled Voltage Source/LConn1
  ERef/LConn1 -- Controlled Voltage Source/RConn2

== system Manipulator_Power_Simulink1/JOINT2/Controller/Speed/Step Rate and Direction/IC Analog Output REV ==
  SL : Inport  RequirementInfo={} %GIDa_debb2f0b_e9db_48ac_a905_bbc09ffd9690
  Controlled Voltage Source : fl_lib/Electrical/Electrical Sources/Controlled Voltage Source  RequirementInfo={} %GIDa_70a46d02_91d6_4f46_a65e_01fd8a877839
  ERef : fl_lib/Electrical/Electrical Elements/Electrical Reference  RequirementInfo={} %GIDa_a5e6cf12_e734_45c2_a779_bd7e474a6343
  Simulink-PS Converter : nesl_utility/Simulink-PS Converter  RequirementInfo={} %GIDa_ad3e4330_6f4e_435e_928f_0196cef58052  PhysicalDomain=network_engine_domain  SubClassName=ps_input  LeftPortType=input  RightPortType=output  PseudoPeriodic=off  Frequencies=[]  NoiseDistribution=none  NoiseParameters=[]  Unit=V  AffineConversion=off  FilteringAndDerivatives=zero  SimscapeFilterOrder=1  InputFilterTimeConstant=.001  UdotUserProvided=0
      settings: SourceProductBaseCode=PW,SS
  V : PMIOPort  RequirementInfo={} %GIDa_7c960050_bf0b_4217_bb06_00b20c40ba68  Side=Right
  wires:
  SL/1 -> Simulink-PS Converter/1
  connections:
  Simulink-PS Converter/RConn1 -- Controlled Voltage Source/RConn1
  V/RConn1 -- Controlled Voltage Source/LConn1
  ERef/LConn1 -- Controlled Voltage Source/RConn2

== system Manipulator_Power_Simulink1/JOINT2/Controller/Speed/Step Rate and Direction/IC Analog Output Vref ==
  SL : Inport  RequirementInfo={} %GIDa_030d79b7_19b5_4f27_9cfa_e4675b5ba13e
  Controlled Voltage Source : fl_lib/Electrical/Electrical Sources/Controlled Voltage Source  RequirementInfo={} %GIDa_56bfab74_d735_46d7_a716_9c843fce4346
  ERef : fl_lib/Electrical/Electrical Elements/Electrical Reference  RequirementInfo={} %GIDa_8c2dfaca_23e4_4ba7_8fa2_ba4ab37927df
  Simulink-PS Converter : nesl_utility/Simulink-PS Converter  RequirementInfo={} %GIDa_8a22039a_2952_4a41_9762_7bb740be6b57  PhysicalDomain=network_engine_domain  SubClassName=ps_input  LeftPortType=input  RightPortType=output  PseudoPeriodic=off  Frequencies=[]  NoiseDistribution=none  NoiseParameters=[]  Unit=V  AffineConversion=off  FilteringAndDerivatives=zero  SimscapeFilterOrder=1  InputFilterTimeConstant=.001  UdotUserProvided=0
      settings: SourceProductBaseCode=PW,SS
  V : PMIOPort  RequirementInfo={} %GIDa_6cdd90ae_2fa4_4905_87fb_25103b3bebe8  Side=Right
  wires:
  SL/1 -> Simulink-PS Converter/1
  connections:
  ERef/LConn1 -- Controlled Voltage Source/RConn2
  V/RConn1 -- Controlled Voltage Source/LConn1
  Simulink-PS Converter/RConn1 -- Controlled Voltage Source/RConn1

== system Manipulator_Power_Simulink1/JOINT3/Controller/Speed/Step Rate and Direction/IC Analog Output REV ==
  SL : Inport  RequirementInfo={} %GIDa_1e6db38e_40dd_4d89_b3b4_5d988e5939ba
  Controlled Voltage Source : fl_lib/Electrical/Electrical Sources/Controlled Voltage Source  RequirementInfo={} %GIDa_7fa239ed_fee5_418e_a728_d25bebc07cfc
  ERef : fl_lib/Electrical/Electrical Elements/Electrical Reference  RequirementInfo={} %GIDa_6ba7f881_c682_4057_b117_42cb9fabd161
  Simulink-PS Converter : nesl_utility/Simulink-PS Converter  RequirementInfo={} %GIDa_e00b56a4_ed81_4d8c_974e_153006573c7f  PhysicalDomain=network_engine_domain  SubClassName=ps_input  LeftPortType=input  RightPortType=output  PseudoPeriodic=off  Frequencies=[]  NoiseDistribution=none  NoiseParameters=[]  Unit=V  AffineConversion=off  FilteringAndDerivatives=zero  SimscapeFilterOrder=1  InputFilterTimeConstant=.001  UdotUserProvided=0
      settings: SourceProductBaseCode=PW,SS
  V : PMIOPort  RequirementInfo={} %GIDa_f1c621ca_9645_4c47_9ef9_e391b6af907c  Side=Right
  wires:
  SL/1 -> Simulink-PS Converter/1
  connections:
  ERef/LConn1 -- Controlled Voltage Source/RConn2
  V/RConn1 -- Controlled Voltage Source/LConn1
  Simulink-PS Converter/RConn1 -- Controlled Voltage Source/RConn1

== system Manipulator_Power_Simulink1/JOINT3/Controller/Speed/Step Rate and Direction/IC Analog Output Vref ==
  SL : Inport  RequirementInfo={} %GIDa_7704a46e_ebd5_4bd6_a9c8_495cf18e6496
  Controlled Voltage Source : fl_lib/Electrical/Electrical Sources/Controlled Voltage Source  RequirementInfo={} %GIDa_0eb777a7_3668_44be_a9ec_cfc53c47363c
  ERef : fl_lib/Electrical/Electrical Elements/Electrical Reference  RequirementInfo={} %GIDa_901adcc9_d447_4fc8_9204_8a67572f5cea
  Simulink-PS Converter : nesl_utility/Simulink-PS Converter  RequirementInfo={} %GIDa_f8a3a55c_696d_472a_8ed7_13b93ec1ef8e  PhysicalDomain=network_engine_domain  SubClassName=ps_input  LeftPortType=input  RightPortType=output  PseudoPeriodic=off  Frequencies=[]  NoiseDistribution=none  NoiseParameters=[]  Unit=V  AffineConversion=off  FilteringAndDerivatives=zero  SimscapeFilterOrder=1  InputFilterTimeConstant=.001  UdotUserProvided=0
      settings: SourceProductBaseCode=PW,SS
  V : PMIOPort  RequirementInfo={} %GIDa_db1be55c_15c7_40dd_b09c_f557ae72fc44  Side=Right
  wires:
  SL/1 -> Simulink-PS Converter/1
  connections:
  Simulink-PS Converter/RConn1 -- Controlled Voltage Source/RConn1
  V/RConn1 -- Controlled Voltage Source/LConn1
  ERef/LConn1 -- Controlled Voltage Source/RConn2

== system Manipulator_Power_Simulink1/JOINT4/Controller/Speed/Step Rate and Direction/IC Analog Output REV ==
  SL : Inport  RequirementInfo={} %GIDa_223ae48a_3124_404c_a70c_f1a67e7abbff
  Controlled Voltage Source : fl_lib/Electrical/Electrical Sources/Controlled Voltage Source  RequirementInfo={} %GIDa_15b38eaf_7740_4c51_8d4d_6ed1dd4eb123
  ERef : fl_lib/Electrical/Electrical Elements/Electrical Reference  RequirementInfo={} %GIDa_0d682834_f452_4942_89ee_40652f2df32b
  Simulink-PS Converter : nesl_utility/Simulink-PS Converter  RequirementInfo={} %GIDa_fb3f1672_871b_41b6_8586_c79f2afa5436  PhysicalDomain=network_engine_domain  SubClassName=ps_input  LeftPortType=input  RightPortType=output  PseudoPeriodic=off  Frequencies=[]  NoiseDistribution=none  NoiseParameters=[]  Unit=V  AffineConversion=off  FilteringAndDerivatives=zero  SimscapeFilterOrder=1  InputFilterTimeConstant=.001  UdotUserProvided=0
      settings: SourceProductBaseCode=PW,SS
  V : PMIOPort  RequirementInfo={} %GIDa_455c06bc_531b_43e8_850e_d1aa99e0971f  Side=Right
  wires:
  SL/1 -> Simulink-PS Converter/1
  connections:
  Simulink-PS Converter/RConn1 -- Controlled Voltage Source/RConn1
  V/RConn1 -- Controlled Voltage Source/LConn1
  ERef/LConn1 -- Controlled Voltage Source/RConn2

== system Manipulator_Power_Simulink1/JOINT4/Controller/Speed/Step Rate and Direction/IC Analog Output Vref ==
  SL : Inport  RequirementInfo={} %GIDa_8e1354b7_d400_4bac_bdac_485d5aefa13b
  Controlled Voltage Source : fl_lib/Electrical/Electrical Sources/Controlled Voltage Source  RequirementInfo={} %GIDa_2d66a91e_0377_48f8_91ce_eb0f5e90987a
  ERef : fl_lib/Electrical/Electrical Elements/Electrical Reference  RequirementInfo={} %GIDa_88bdde4c_a278_40f1_b7dc_8b7952c2a77f
  Simulink-PS Converter : nesl_utility/Simulink-PS Converter  RequirementInfo={} %GIDa_96106f1f_e816_49bb_b31d_ff6022300ee6  PhysicalDomain=network_engine_domain  SubClassName=ps_input  LeftPortType=input  RightPortType=output  PseudoPeriodic=off  Frequencies=[]  NoiseDistribution=none  NoiseParameters=[]  Unit=V  AffineConversion=off  FilteringAndDerivatives=zero  SimscapeFilterOrder=1  InputFilterTimeConstant=.001  UdotUserProvided=0
      settings: SourceProductBaseCode=PW,SS
  V : PMIOPort  RequirementInfo={} %GIDa_c0dbc115_34b3_4bde_bc6d_7dac7f6af86a  Side=Right
  wires:
  SL/1 -> Simulink-PS Converter/1
  connections:
  ERef/LConn1 -- Controlled Voltage Source/RConn2
  V/RConn1 -- Controlled Voltage Source/LConn1
  Simulink-PS Converter/RConn1 -- Controlled Voltage Source/RConn1
